simulink model "InvertedPendulum_PID"  (R2015b)
settings: Solver=FixedStepAuto  StartTime=0.0  StopTime=simtime  FixedStep=1/30  RelTol=1e-3
values from neighbouring files (symbols this model uses):
  b = 0.01    [inverted_pendulum.m]    (also in inverted_pendulum_controlled.m)
  d = 0.02    [inverted_pendulum.m]    (also in inverted_pendulum_controlled.m)
  F2 = 0    [inverted_pendulum.m]    (also in inverted_pendulum_controlled.m = -1)
  F2_time = 0    [inverted_pendulum.m]    (also in inverted_pendulum_controlled.m = 4)
  g = 9.82    [inverted_pendulum.m]    (also in inverted_pendulum_controlled.m)
  l = 0.3    [inverted_pendulum.m]    (also in inverted_pendulum_controlled.m)
  m = 0.2    [inverted_pendulum.m]    (also in inverted_pendulum_controlled.m)
  M = 0.5    [inverted_pendulum.m]    (also in inverted_pendulum_controlled.m)
  ref = 0    [inverted_pendulum_controlled.m]
  theta_init = pi/6    (= 0.523598775598)    [inverted_pendulum.m]    (also in inverted_pendulum_controlled.m = 0.2)
libraries: simulink x1
settings Model: Creator=Andreas  LastModifiedBy=Andreas

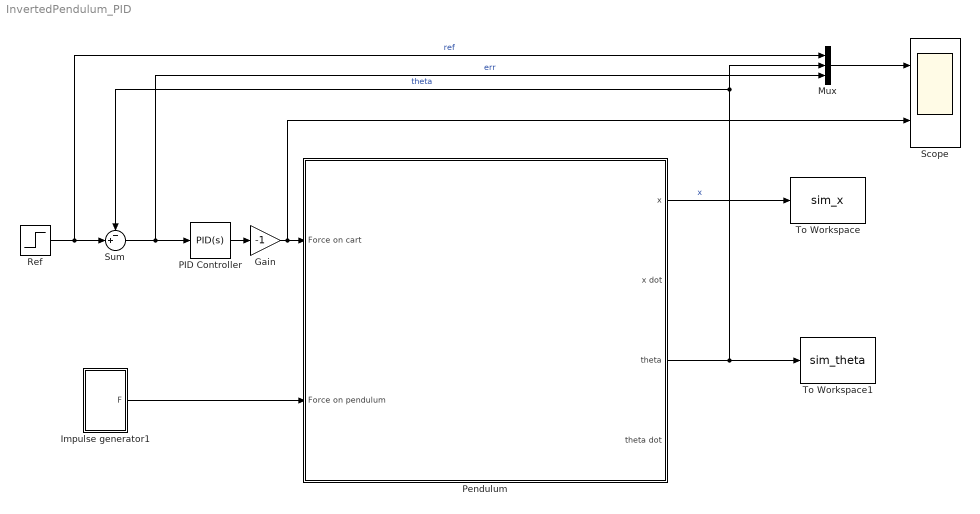
== system InvertedPendulum_PID ==
  Gain : Gain  Gain=-1
  Impulse generator1 : Subsystem
  Mux : Mux  Inputs=3
  PID Controller : simulink/Continuous/PID Controller  Controller=PID  TimeDomain=Continuous-time  SampleTime=-1  IntegratorMethod=Forward Euler  FilterMethod=Forward Euler  Form=Parallel  UseFilter=on  ControllerParametersSource=internal  P=50  I=1  D=0  N=100  InitialConditionSource=internal  InitialConditionForIntegrator=0  InitialConditionForFilter=0  ExternalReset=none  LimitOutput=off  UpperSaturationLimit=inf  LowerSaturationLimit=-inf  LinearizeAsGain=on  AntiWindupMode=none  Kb=1  TrackingMode=off  Kt=1  PParamMin=[]  PParamMax=[]  IParamMin=[]  IParamMax=[]  DParamMin=[]  DParamMax=[]  NParamMin=[]  NParamMax=[]  KbParamMin=[]  KbParamMax=[]  KtParamMin=[]  KtParamMax=[]  POutMin=[]  POutMax=[]  IOutMin=[]  IOutMax=[]  DOutMin=[]  DOutMax=[]  NOutMin=[]  NOutMax=[]  KbOutMin=[]  KbOutMax=[]  KtOutMin=[]  KtOutMax=[]  IntegratorOutMin=[]  IntegratorOutMax=[]  FilterOutMin=[]  FilterOutMax=[]  SumOutMin=[]  SumOutMax=[]  SumI1OutMin=[]  SumI1OutMax=[]  SumI2OutMin=[]  SumI2OutMax=[]  SumI3OutMin=[]  SumI3OutMax=[]  SumDOutMin=[]  SumDOutMax=[]  SaturationOutMin=[]  SaturationOutMax=[]  IntegratorContinuousStateAttributes=''  IntegratorStateMustResolveToSignalObject=off  IntegratorRTWStateStorageClass=Auto  FilterContinuousStateAttributes=''  FilterStateMustResolveToSignalObject=off  FilterRTWStateStorageClass=Auto  DifferentiatorICPrevScaledInput=0  DifferentiatorOutMin=[]  DifferentiatorOutMax=[]
  Pendulum : Subsystem
      mask Display:
      | image('invpend.jpg')
      | port_label('input', 1, 'Force on cart')
      | port_label('input', 2, 'Force on pendulum')
      | port_label('output', 1, 'x')
      | port_label('output', 2, 'x dot')
      | port_label('output', 3, 'theta')
      | port_label('output', 4, 'theta dot')
  Ref : Step  Time=0  After=ref  SampleTime=0
  Scope : Scope  NumInputPorts=2
  Sum : Sum  Inputs=-+|
  To Workspace : ToWorkspace  VariableName=sim_x  SaveFormat=Timeseries  SampleTime=-1
  To Workspace1 : ToWorkspace  VariableName=sim_theta  SaveFormat=Timeseries  SampleTime=-1
  wires:
  Impulse generator1/1(F) -> Pendulum/2(Force on pendulum)
  Pendulum/1("x ") -> To Workspace/1  "x"
  Pendulum/3(theta) -> Mux/2, Sum/1, To Workspace1/1  "theta"
  Ref/1 -> Mux/1, Sum/2  "ref"
  Sum/1 -> Mux/3, PID Controller/1  "err"
  PID Controller/1 -> Gain/1
  Gain/1 -> Scope/2, Pendulum/1(Force on cart)
  Mux/1 -> Scope/1

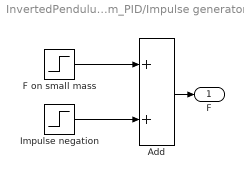
== system InvertedPendulum_PID/Impulse generator1 ==
  Add : Sum
  F on small mass : Step  Time=F2_time  After=F2  SampleTime=0
  Impulse negation : Step  Time=F2_time+0.1  After=-F2  SampleTime=0
  F : Outport
  wires:
  Add/1 -> F/1
  F on small mass/1 -> Add/1
  Impulse negation/1 -> Add/2

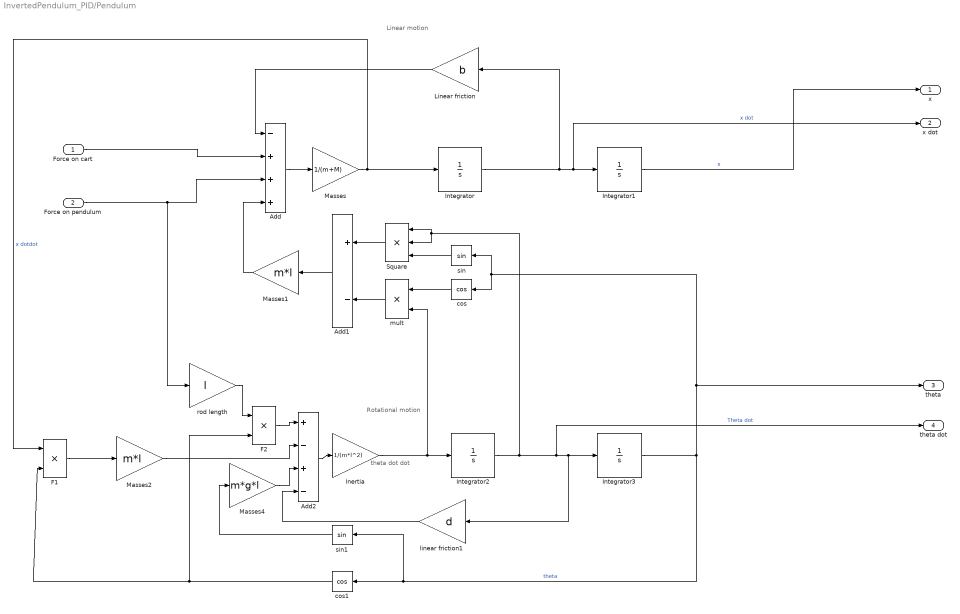
== system InvertedPendulum_PID/Pendulum ==
  note: theta dot dot
  note: Linear motion
  note: Rotational motion
  Force on cart : Inport
  Force on pendulum : Inport  Port=2
  Add : Sum  Inputs=-+++
  Add1 : Sum  Inputs=+-
  Add2 : Sum  Inputs=+-+-
  F1 : Product
  F2 : Product
  Inertia : Gain  Gain=1/(m*l^2)
  Integrator : Integrator
  Integrator1 : Integrator
  Integrator2 : Integrator
  Integrator3 : Integrator  InitialCondition=theta_init
  Linear friction : Gain  Gain=b
  Masses : Gain  Gain=1/(m+M)
  Masses1 : Gain  Gain=m*l
  Masses2 : Gain  Gain=m*l
  Masses4 : Gain  Gain=m*g*l
  Square : Product  Inputs=3
  cos : Trigonometry  Operator=cos
  cos1 : Trigonometry  Operator=cos
  linear friction1 : Gain  Gain=d
  mult : Product
  rod length : Gain  Gain=l
  sin : Trigonometry
  sin1 : Trigonometry
  "x " : Outport
  x dot : Outport  Port=2
  theta : Outport  Port=3
  theta dot : Outport  Port=4
  wires:
  Integrator1/1 -> "x "/1  "x"
  linear friction1/1 -> Add2/4
  Force on cart/1 -> Add/2
  Masses/1 -> F1/1, Integrator/1  "x dotdot"
  Add/1 -> Masses/1
  F2/1 -> Add2/1
  F1/1 -> Masses2/1
  Integrator3/1 -> sin1/1, cos1/1, cos/1, sin/1, theta/1  "theta"
  cos1/1 -> F2/2, F1/2
  Linear friction/1 -> Add/1
  Add1/1 -> Masses1/1
  mult/1 -> Add1/2
  Masses1/1 -> Add/4
  sin/1 -> Square/3
  Integrator2/1 -> Square/2, Square/1, theta dot/1, linear friction1/1, Integrator3/1  "Theta dot"
  Inertia/1 -> mult/2, Integrator2/1
  Integrator/1 -> Linear friction/1, x dot/1, Integrator1/1  "x dot"
  Add2/1 -> Inertia/1
  Force on pendulum/1 -> Add/3, rod length/1
  Square/1 -> Add1/1
  sin1/1 -> Masses4/1
  Masses4/1 -> Add2/3
  cos/1 -> mult/1
  rod length/1 -> F2/1
  Masses2/1 -> Add2/2
